simulink model "plantlib"  (Simulink 6.2)
settings: Solver=ode45  SolverMode=SingleTasking  StartTime=0.0  StopTime=999999  MaxStep=10  RelTol=1e-3  AbsTol=1e-3
settings Model: Creator=jacobs  LastModifiedBy=jacobs  ExtModeAutoUpdateStatusClock=off
settings DataIOCC: LimitDataPoints=off  SaveOutput=off  SaveTime=off
settings OptimizationCC: BlockReduction=off  BooleanDataType=off
settings HardwareCC: TargetUnknown=on
settings STFCustomTargetCC: TargetFcnLib=ansi_tfl_tmw.mat  GenFloatMathFcnCalls=ANSI_C  ModelReferenceCompliant=off  SystemTargetFile=grt.tlc

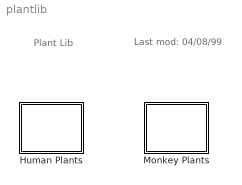
== system plantlib ==
  note: Plant Lib
  note: Last mod:
      | 04/08/99
  Human Plants : Subsystem
      mask Display: disp('Human\nPlants')
  Monkey Plants : Subsystem
      mask Display: disp('Monkey\nPlants')

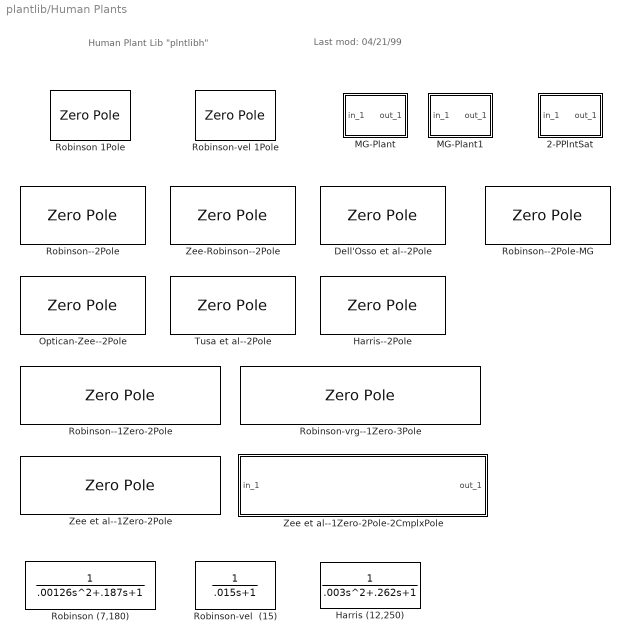
== system plantlib/Human Plants ==
  note: Last mod:
      | 04/21/99
  note: Human Plant Lib
      | "plntlibh"
  2-PPlntSat : Subsystem
      mask Display: disp('2-P Plant\n[Sat]')
  Dell'Osso et al--2Pole : ZeroPole  Zeros=[ ]  Poles=[ -1/.007 -1/.150]  Gain=[(1/.007)*(1/.150)]
  Harris (12,250) : TransferFcn  Denominator=[.003 .262 1]
  Harris--2Pole : ZeroPole  Zeros=[ ]  Poles=[ -1/.012 -1/.250]  Gain=[(1/.012)*(1/.250)]
  MG-Plant : Subsystem
      mask Display: disp('MG Plant\n[K,tau,sat]')
  MG-Plant1 : Subsystem
      mask Display: disp('MG Plant\n[K,tau,sat]')
  Optican-Zee--2Pole : ZeroPole  Zeros=[ ]  Poles=[ -1/.015-1/.100]  Gain=[(1/.015)*(1/.100)]
  Robinson 1Pole : ZeroPole  Zeros=[ ]  Poles=[ -1/.250]  Gain=[(1/.250)]
  Robinson (7,180) : TransferFcn  Denominator=[.00126 .187 1]
  Robinson--1Zero-2Pole : ZeroPole  Zeros=[-1/.020]  Poles=[-1/.012 -1/.285]  Gain=[(.020)*(1/.012)*(1/.285)]
  Robinson--2Pole : ZeroPole  Zeros=[ ]  Poles=[ -1/.007 -1/.180]  Gain=[(1/.007)*(1/.180)]
  Robinson--2Pole-MG : ZeroPole  Zeros=[ ]  Poles=[ -1/.007 -1/.180]  Gain=[(1/.007)*(1/.180)]*0.5
  Robinson-vel  (15) : TransferFcn  Denominator=[.015 1]
  Robinson-vel 1Pole : ZeroPole  Zeros=[ ]  Poles=[ -1/.015]  Gain=[(1/.015)]
  Robinson-vrg--1Zero-3Pole : ZeroPole  Zeros=[-1/.020]  Poles=[-1/.0083 -1/.285 -1/.5]  Gain=[(.020)*(1/.0083)*(1/.285)*(1/.5)]
  Tusa et al--2Pole : ZeroPole  Zeros=[ ]  Poles=[ -1/.010-1/.150]  Gain=[(1/.010)*(1/.150)]
  Zee et al--1Zero-2Pole : ZeroPole  Zeros=[-1/.080]  Poles=[-1/.012 -1/.300]  Gain=[(.080)*(1/.012)*(1/.300)]
  Zee et al--1Zero-2Pole-2CmplxPole : Subsystem
      mask Display: disp('(.080)*(1/.010)*(1/.300)*40000(s+1/.080)\n----------------------------------------------------------\n(s+1/.010)(s+1/.300)(s2+240s+40000)')
  Zee-Robinson--2Pole : ZeroPole  Zeros=[ ]  Poles=[ -1/.012 -1/.150]  Gain=[(1/.012)*(1/.150)]

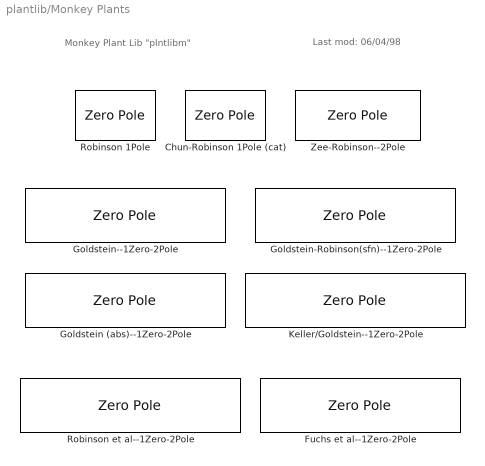
== system plantlib/Monkey Plants ==
  note: Monkey Plant Lib
      | "plntlibm"
  note: Last mod:
      | 06/04/98
  Chun-Robinson 1Pole (cat) : ZeroPole  Zeros=[ ]  Poles=[ -1/.200]  Gain=[(1/.200)]
  Fuchs et al--1Zero-2Pole : ZeroPole  Zeros=[-1/.140]  Poles=[-1/.012 -1/.260]  Gain=[(.140)*(1/.012)*(1/.260)]
  Goldstein (abs)--1Zero-2Pole : ZeroPole  Zeros=[-1/.100]  Poles=[-1/.012 -1/.200]  Gain=[(.100)*(1/.012)*(1/.200)]
  Goldstein--1Zero-2Pole : ZeroPole  Zeros=[-1/.068]  Poles=[-1/.012 -1/.180]  Gain=[(.068)*(1/.012)*(1/.180)]
  Goldstein-Robinson(sfn)--1Zero-2Pole : ZeroPole  Zeros=[-1/.090]  Poles=[-1/.020 -1/.170]  Gain=[(.090)*(1/.020)*(1/.170)]
  Keller/Goldstein--1Zero-2Pole : ZeroPole  Zeros=[-1/.072]  Poles=[-1/.012 -1/.260]  Gain=[(.072)*(1/.012)*(1/.260)]
  Robinson 1Pole : ZeroPole  Zeros=[ ]  Poles=[ -1/.160]  Gain=[(1/.160)]
  Robinson et al--1Zero-2Pole : ZeroPole  Zeros=[-1/.092]  Poles=[-1/.012 -1/.260]  Gain=[(.092)*(1/.012)*(1/.260)]
  Zee-Robinson--2Pole : ZeroPole  Zeros=[ ]  Poles=[ -1/.012 -1/.150]  Gain=[(1/.012)*(1/.150)]

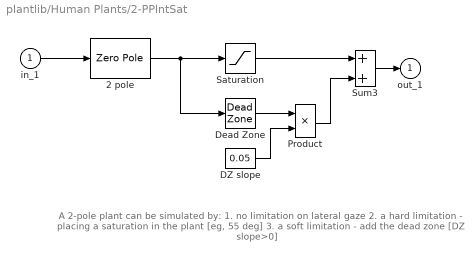
== system plantlib/Human Plants/2-PPlntSat ==
  note: A 2-pole plant can be simulated by:
      | 1. no limitation on lateral gaze
      | 2. a hard limitation - placing a saturation in the plant [eg, 55 deg]
      | 3. a soft limitation - add the dead zone  [DZ slope>0]
  in_1 : Inport  Port=1  LatchInput=off
  2 pole : ZeroPole  Zeros=[ ]  Poles=[ -1/.18 -1/.007]  Gain=[1/.18 * 1/.007]
      mask Display: disp('2-pole\nPlant')
  DZ slope : Constant  Value=0.05
  Dead Zone : DeadZone  LowerValue=-55  UpperValue=55  SaturateOnIntegerOverflow=on
  Product : Product  SaturateOnIntegerOverflow=on  RndMeth=Zero  InputSameDT=on
  Saturation : Saturate  UpperLimit=55  LowerLimit=-55
  Sum3 : Sum  SaturateOnIntegerOverflow=on  InputSameDT=on
  out_1 : Outport  InitialOutput=0
  wires:
  in_1/1 -> 2 pole/1
  2 pole/1 -> Dead Zone/1, Saturation/1
  Dead Zone/1 -> Product/1
  Saturation/1 -> Sum3/1
  Sum3/1 -> out_1/1
  Product/1 -> Sum3/2
  DZ slope/1 -> Product/2

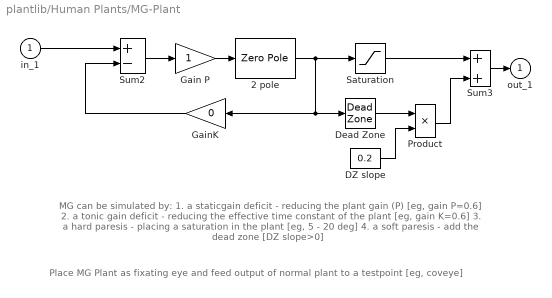
== system plantlib/Human Plants/MG-Plant ==
  note: MG can be simulated by:
      | 1. a staticgain deficit -  reducing the plant gain (P) [eg, gain P=0.6]
      | 2. a tonic gain deficit - reducing the effective time constant of the plant [eg, gain K=0.6]
      | 3. a hard paresis - placing a saturation in the plant [eg, 5 - 20 deg]
      | 4. a soft paresis - add the dead zone  [DZ slope>0]
  note: Place MG Plant as fixating eye and feed output of normal plant to a testpoint [eg, coveye]
  in_1 : Inport  Port=1  LatchInput=off
  2 pole : ZeroPole  Zeros=[ ]  Poles=[ -1/.18 -1/.007]  Gain=[1/.18 * 1/.007]
      mask Display: disp('2-pole\nPlant')
  DZ slope : Constant  Value=0.2
  Dead Zone : DeadZone  LowerValue=-5  UpperValue=5  SaturateOnIntegerOverflow=on
  Gain P : Gain  SaturateOnIntegerOverflow=on
  GainK : Gain  Orientation=left  Gain=0  SaturateOnIntegerOverflow=on
  Product : Product  SaturateOnIntegerOverflow=on  RndMeth=Zero  InputSameDT=on
  Saturation : Saturate  UpperLimit=5  LowerLimit=-5
  Sum2 : Sum  Inputs=+-  SaturateOnIntegerOverflow=on  InputSameDT=on
  Sum3 : Sum  SaturateOnIntegerOverflow=on  InputSameDT=on
  out_1 : Outport  InitialOutput=0
  wires:
  DZ slope/1 -> Product/2
  Product/1 -> Sum3/2
  Sum3/1 -> out_1/1
  Saturation/1 -> Sum3/1
  Dead Zone/1 -> Product/1
  2 pole/1 -> Dead Zone/1, GainK/1, Saturation/1
  Gain P/1 -> 2 pole/1
  Sum2/1 -> Gain P/1
  in_1/1 -> Sum2/1
  GainK/1 -> Sum2/2

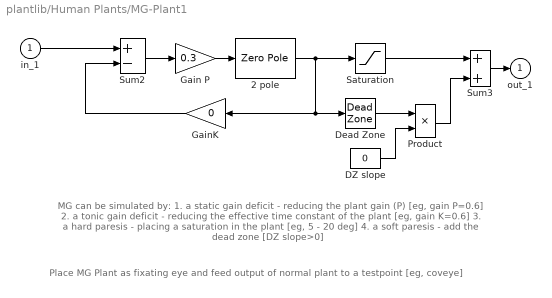
== system plantlib/Human Plants/MG-Plant1 ==
  note: MG can be simulated by:
      | 1. a static gain deficit -  reducing the plant gain (P) [eg, gain P=0.6]
      | 2. a tonic gain deficit - reducing the effective time constant of the plant [eg, gain K=0.6]
      | 3. a hard paresis - placing a saturation in the plant [eg, 5 - 20 deg]
      | 4. a soft paresis - add the dead zone  [DZ slope>0]
  note: Place MG Plant as fixating eye and feed output of normal plant to a testpoint [eg, coveye]
  in_1 : Inport  Port=1  LatchInput=off
  2 pole : ZeroPole  Zeros=[ ]  Poles=[ -1/.18 -1/.007]  Gain=[1/.18 * 1/.007]
      mask Display: disp('2-pole\nPlant')
  DZ slope : Constant  Value=0
  Dead Zone : DeadZone  LowerValue=-5  UpperValue=12  SaturateOnIntegerOverflow=on
  Gain P : Gain  Gain=0.3  SaturateOnIntegerOverflow=on
  GainK : Gain  Orientation=left  Gain=0  SaturateOnIntegerOverflow=on
  Product : Product  SaturateOnIntegerOverflow=on  RndMeth=Zero  InputSameDT=on
  Saturation : Saturate  UpperLimit=50  LowerLimit=-50
  Sum2 : Sum  Inputs=+-  SaturateOnIntegerOverflow=on  InputSameDT=on
  Sum3 : Sum  SaturateOnIntegerOverflow=on  InputSameDT=on
  out_1 : Outport  InitialOutput=0
  wires:
  DZ slope/1 -> Product/2
  Product/1 -> Sum3/2
  Sum3/1 -> out_1/1
  Saturation/1 -> Sum3/1
  Dead Zone/1 -> Product/1
  2 pole/1 -> Dead Zone/1, GainK/1, Saturation/1
  Gain P/1 -> 2 pole/1
  Sum2/1 -> Gain P/1
  in_1/1 -> Sum2/1
  GainK/1 -> Sum2/2

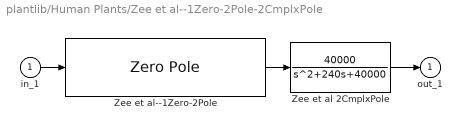
== system plantlib/Human Plants/Zee et al--1Zero-2Pole-2CmplxPole ==
  in_1 : Inport  Port=1  LatchInput=off
  Zee et al 2CmplxPole : TransferFcn  Numerator=[40000]  Denominator=[1 240 40000]
  Zee et al--1Zero-2Pole : ZeroPole  Zeros=[-1/.080]  Poles=[-1/.012 -1/.300]  Gain=[(.080)*(1/.012)*(1/.300)]
  out_1 : Outport  InitialOutput=0
  wires:
  in_1/1 -> Zee et al--1Zero-2Pole/1
  Zee et al 2CmplxPole/1 -> out_1/1
  Zee et al--1Zero-2Pole/1 -> Zee et al 2CmplxPole/1
